simulink model "controlled_motorcycle_plant"  (R2018b)
settings: Solver=VariableStepAuto  StartTime=0.0  StopTime=10.0  RelTol=1e-3
values from neighbouring files (symbols this model uses):
  v = 50/3.6    (= 13.8888888889)    [parameters.m]
libraries: dspsrcs4 x1
settings Model: Creator=Master Broda  LastModifiedBy=Master Broda

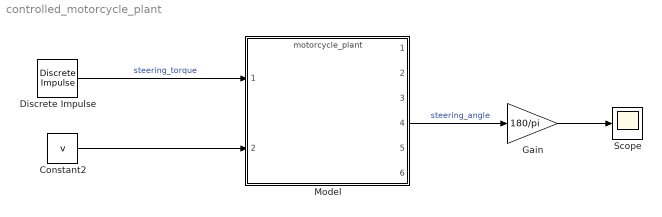
== system controlled_motorcycle_plant ==
  Constant2 : Constant  Value=v
  Discrete Impulse : dspsrcs4/Discrete  Impulse  Delay=0  SampleTime=1  FrameSample=1  OutputFrames=off  dataType=double  isSigned=on  wordLen=16  udDataType=sfix(16)  fracBitsMode=Best precision  numFracBits=15  OutDataTypeStr=double  LastOutDataTypeStr=double
  Gain : Gain  Gain=180/pi
  Model : ModelReference  ModelNameDialog=motorcycle_plant.slx  SimulationMode=Normal  ModelReferenceVersion=1.17
  Scope : Scope
  wires:
  Discrete Impulse/1 -> Model/1  "steering_torque"
  Model/4 -> Gain/1  "steering_angle"
  Constant2/1 -> Model/2
  Gain/1 -> Scope/1
